simulink model "engine_throttle_control_eric_2"  (R2026a)
settings: Solver=VariableStepAuto
undefined symbols (not defined in the file or in its folder): constantsSTADPOLE
settings Model: Creator=Eric  LastModifiedBy=Eric

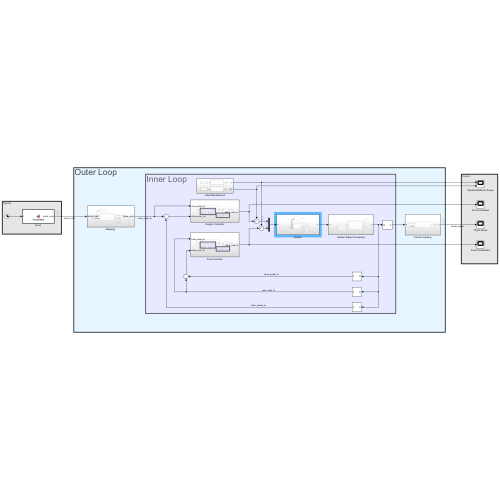
[thumbnail: Simulink's stored preview of the top-level diagram]
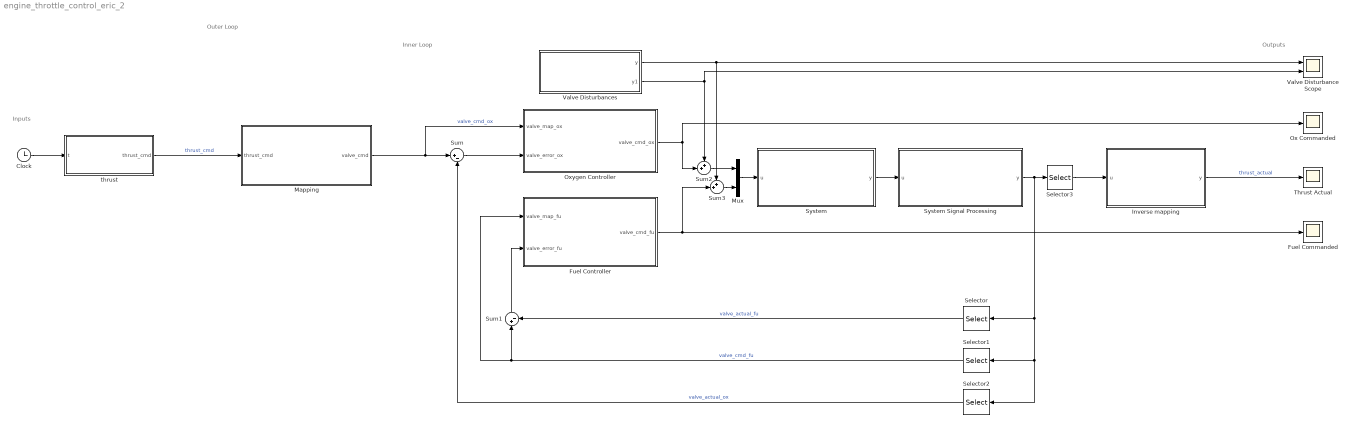
== system engine_throttle_control_eric_2 ==
  note: Inputs
  note: Outputs
  note: Outer Loop
  note: Inner Loop
  Clock : Clock
  Fuel Commanded : Scope
      settings: ActiveDisplayYMinimum=10.461022120017061  ActiveDisplayYMaximum=85.850800919846463  DataLoggingVariableName=ScopeData2
  Fuel Controller : Subsystem
  Inverse mapping : Subsystem
  Mapping : Subsystem
  Mux : Mux  Inputs=2
  Ox Commanded : Scope
      settings: ActiveDisplayYMinimum=6.6145825944924042  ActiveDisplayYMaximum=206.61458259449239  DataLoggingVariableName=ScopeData3
  Oxygen Controller : Subsystem
  Selector : Selector  InputPortWidth=6  IndexOptions=Index vector (dialog)  Indices=4  OutputSizes=1
  Selector1 : Selector  InputPortWidth=6  IndexOptions=Index vector (dialog)  Indices=3  OutputSizes=1
  Selector2 : Selector  InputPortWidth=6  IndexOptions=Index vector (dialog)  Indices=2  OutputSizes=1
  Selector3 : Selector  InputPortWidth=6  IndexOptions=Index vector (dialog)  Indices=1  OutputSizes=1
  Sum : Sum  Inputs=|+-
  Sum1 : Sum  Inputs=|+-
  Sum2 : Sum  Inputs=++|
  Sum3 : Sum  Inputs=++|
  System : Subsystem
  System Signal Processing : Subsystem
  Thrust Actual : Scope
      settings: ActiveDisplayYMinimum=-315.35197548585552  ActiveDisplayYMaximum=2620.6061100786883
  Valve Disturbance Scope : Scope  NumInputPorts=2
      settings: ActiveDisplayYMinimum=-2.4231337070144896  ActiveDisplayYMaximum=3.2939078653946221
  Valve Disturbances : Subsystem
  thrust : MATLAB Function  TreatAsAtomicUnit=on
  wires:
  Clock/1 -> thrust/1(t)
  Inverse mapping/1(y) -> Thrust Actual/1  "thrust_actual"
  thrust/1(thrust_cmd) -> Mapping/1(thrust_cmd)  "thrust_cmd"
  Sum/1 -> Oxygen Controller/2(valve_error_ox)
  Mapping/1(valve_cmd) -> Sum/1, Oxygen Controller/1(valve_map_ox)  "valve_cmd_ox"
  Oxygen Controller/1(valve_cmd_ox) -> Ox Commanded/1, Sum2/2
  System/1(y) -> System Signal Processing/1(u)
  System Signal Processing/1(y) -> Selector/1, Selector1/1, Selector2/1, Selector3/1
  Sum1/1 -> Fuel Controller/2(valve_error_fu)
  Fuel Controller/1(valve_cmd_fu) -> Sum3/2, Fuel Commanded/1
  Selector/1 -> Sum1/2  "valve_actual_fu"
  Selector1/1 -> Sum1/1, Fuel Controller/1(valve_map_fu)  "valve_cmd_fu"
  Selector2/1 -> Sum/2  "valve_actual_ox"
  Selector3/1 -> Inverse mapping/1(u)
  Sum2/1 -> Mux/1
  Valve Disturbances/2(y1) -> Sum2/1, Valve Disturbance Scope/2
  Sum3/1 -> Mux/2
  Valve Disturbances/1(y) -> Sum3/1, Valve Disturbance Scope/1
  Mux/1 -> System/1(u)

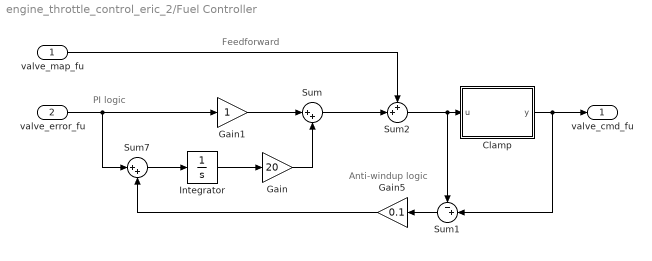
== system engine_throttle_control_eric_2/Fuel Controller ==
  note: PI logic
  note: Anti-windup logic
  note: Feedforward
  valve_map_fu : Inport
  valve_error_fu : Inport  Port=2
  Clamp : MATLAB Function  TreatAsAtomicUnit=on
  Gain : Gain  Gain=20
  Gain1 : Gain
  Gain5 : Gain  Gain=0.1
  Integrator : Integrator
  Sum : Sum  Inputs=|++
  Sum1 : Sum  Inputs=-+|
  Sum2 : Sum  Inputs=++|
  Sum7 : Sum  Inputs=|++
  valve_cmd_fu : Outport
  wires:
  Sum2/1 -> Clamp/1(u), Sum1/1
  Clamp/1(y) -> valve_cmd_fu/1, Sum1/2
  valve_map_fu/1 -> Sum2/1
  Sum1/1 -> Gain5/1
  Sum7/1 -> Integrator/1
  valve_error_fu/1 -> Sum7/1, Gain1/1
  Gain5/1 -> Sum7/2
  Gain/1 -> Sum/2
  Gain1/1 -> Sum/1
  Sum/1 -> Sum2/2
  Integrator/1 -> Gain/1

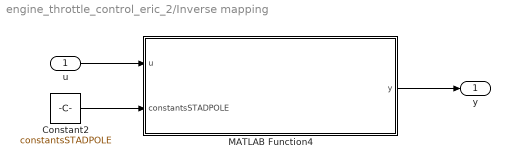
== system engine_throttle_control_eric_2/Inverse mapping ==
  u : Inport
  Constant2 : Constant  Value=constantsSTADPOLE  OutDataTypeStr=Bus: slBus1
  MATLAB Function4 : MATLAB Function  TreatAsAtomicUnit=on
  y : Outport
  wires:
  MATLAB Function4/1(y) -> y/1
  u/1 -> MATLAB Function4/1(u)
  Constant2/1 -> MATLAB Function4/2(constantsSTADPOLE)

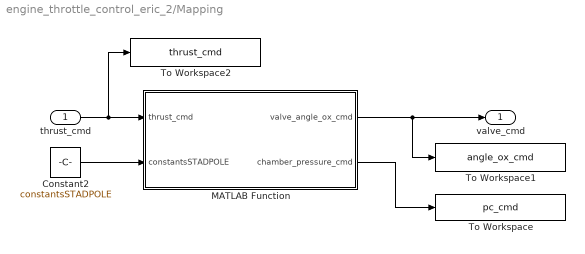
== system engine_throttle_control_eric_2/Mapping ==
  thrust_cmd : Inport
  Constant2 : Constant  Value=constantsSTADPOLE  OutDataTypeStr=Bus: slBus1
  MATLAB Function : MATLAB Function  TreatAsAtomicUnit=on
  To Workspace : ToWorkspace  VariableName=pc_cmd  SaveFormat=Timeseries  SampleTime=-1
  To Workspace1 : ToWorkspace  VariableName=angle_ox_cmd  SaveFormat=Timeseries  SampleTime=-1
  To Workspace2 : ToWorkspace  VariableName=thrust_cmd  SaveFormat=Timeseries  SampleTime=-1
  valve_cmd : Outport
  wires:
  MATLAB Function/1(valve_angle_ox_cmd) -> To Workspace1/1, valve_cmd/1
  thrust_cmd/1 -> To Workspace2/1, MATLAB Function/1(thrust_cmd)
  Constant2/1 -> MATLAB Function/2(constantsSTADPOLE)
  MATLAB Function/2(chamber_pressure_cmd) -> To Workspace/1

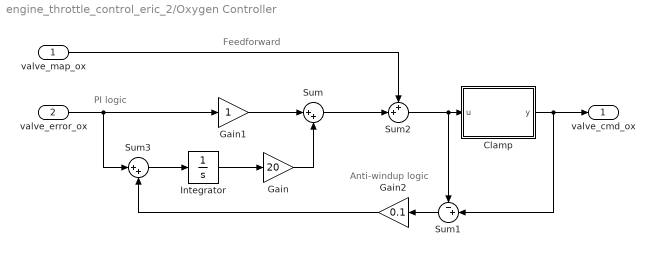
== system engine_throttle_control_eric_2/Oxygen Controller ==
  note: PI logic
  note: Anti-windup logic
  note: Feedforward
  valve_map_ox : Inport
  valve_error_ox : Inport  Port=2
  Clamp : MATLAB Function  TreatAsAtomicUnit=on
  Gain : Gain  Gain=20
  Gain1 : Gain
  Gain2 : Gain  Gain=0.1
  Integrator : Integrator
  Sum : Sum  Inputs=|++
  Sum1 : Sum  Inputs=-+|
  Sum2 : Sum  Inputs=++|
  Sum3 : Sum  Inputs=|++
  valve_cmd_ox : Outport
  wires:
  valve_error_ox/1 -> Sum3/1, Gain1/1
  Integrator/1 -> Gain/1
  Gain1/1 -> Sum/1
  Gain/1 -> Sum/2
  valve_map_ox/1 -> Sum2/1
  Sum3/1 -> Integrator/1
  Sum1/1 -> Gain2/1
  Gain2/1 -> Sum3/2
  Sum/1 -> Sum2/2
  Sum2/1 -> Clamp/1(u), Sum1/1
  Clamp/1(y) -> Sum1/2, valve_cmd_ox/1

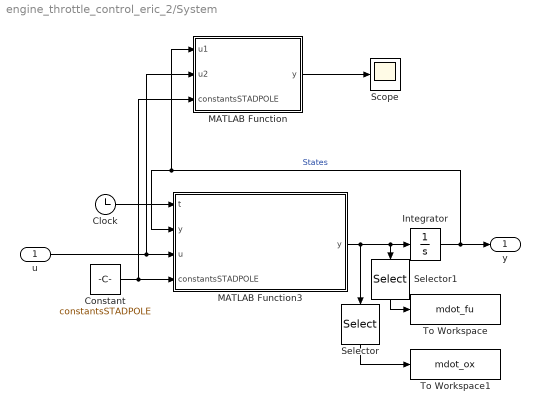
== system engine_throttle_control_eric_2/System ==
  u : Inport
  Clock : Clock
  Constant : Constant  Value=constantsSTADPOLE  OutDataTypeStr=Bus: slBus1
  Integrator : Integrator  InitialCondition=constantsSTADPOLE.init_cond
  MATLAB Function : MATLAB Function  TreatAsAtomicUnit=on
  MATLAB Function3 : MATLAB Function  TreatAsAtomicUnit=on
  Scope : Scope
      settings: DataLoggingVariableName=ScopeData4
  Selector : Selector  InputPortWidth=7  IndexOptions=Index vector (dialog)  Indices=1  OutputSizes=1
  Selector1 : Selector  InputPortWidth=7  IndexOptions=Index vector (dialog)  Indices=2  OutputSizes=1
  To Workspace : ToWorkspace  VariableName=mdot_fu  SaveFormat=Timeseries  SampleTime=-1
  To Workspace1 : ToWorkspace  VariableName=mdot_ox  SaveFormat=Timeseries  SampleTime=-1
  y : Outport
  wires:
  MATLAB Function3/1(y) -> Selector/1, Selector1/1, Integrator/1
  u/1 -> MATLAB Function/2(u2), MATLAB Function3/3(u)
  Integrator/1 -> MATLAB Function3/2("y "), MATLAB Function/1(u1), y/1  "States"
  Constant/1 -> MATLAB Function/3(constantsSTADPOLE), MATLAB Function3/4(constantsSTADPOLE)
  Clock/1 -> MATLAB Function3/1(t)
  Selector/1 -> To Workspace1/1
  Selector1/1 -> To Workspace/1
  MATLAB Function/1(y) -> Scope/1

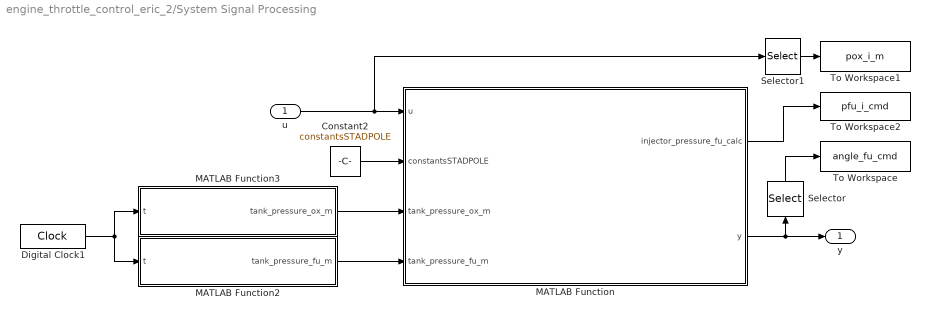
== system engine_throttle_control_eric_2/System Signal Processing ==
  u : Inport
  Constant2 : Constant  Value=constantsSTADPOLE  OutDataTypeStr=Bus: slBus1
  Digital Clock1 : DigitalClock
  MATLAB Function : MATLAB Function  TreatAsAtomicUnit=on
  MATLAB Function2 : MATLAB Function  TreatAsAtomicUnit=on
  MATLAB Function3 : MATLAB Function  TreatAsAtomicUnit=on
  Selector : Selector  InputPortWidth=6  IndexOptions=Index vector (dialog)  Indices=3  OutputSizes=1
  Selector1 : Selector  InputPortWidth=7  IndexOptions=Index vector (dialog)  Indices=4  OutputSizes=1
  To Workspace : ToWorkspace  VariableName=angle_fu_cmd  SaveFormat=Timeseries  SampleTime=-1
  To Workspace1 : ToWorkspace  VariableName=pox_i_m  SaveFormat=Timeseries  SampleTime=-1
  To Workspace2 : ToWorkspace  VariableName=pfu_i_cmd  SaveFormat=Timeseries  SampleTime=-1
  y : Outport
  wires:
  MATLAB Function/2(y) -> y/1, Selector/1
  Constant2/1 -> MATLAB Function/2(constantsSTADPOLE)
  MATLAB Function3/1(tank_pressure_ox_m) -> MATLAB Function/3(tank_pressure_ox_m)
  Digital Clock1/1 -> MATLAB Function3/1(t), MATLAB Function2/1(t)
  MATLAB Function2/1(tank_pressure_fu_m) -> MATLAB Function/4(tank_pressure_fu_m)
  Selector/1 -> To Workspace/1
  Selector1/1 -> To Workspace1/1
  u/1 -> Selector1/1, MATLAB Function/1(u)
  MATLAB Function/1(injector_pressure_fu_calc) -> To Workspace2/1

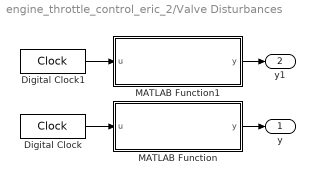
== system engine_throttle_control_eric_2/Valve Disturbances ==
  Digital Clock : DigitalClock
  Digital Clock1 : DigitalClock
  MATLAB Function : MATLAB Function  TreatAsAtomicUnit=on
  MATLAB Function1 : MATLAB Function  TreatAsAtomicUnit=on
  y : Outport
  y1 : Outport  Port=2
  wires:
  MATLAB Function/1(y) -> y/1
  Digital Clock/1 -> MATLAB Function/1(u)
  MATLAB Function1/1(y) -> y1/1
  Digital Clock1/1 -> MATLAB Function1/1(u)

== matlab function engine_throttle_control_eric_2/Fuel Controller/Clamp ==
  data: u input; y output
function y = sat(u)

if u < 0
    y = 0;

elseif 90 < u
    y = 90;

else
    y = u;

end

== matlab function engine_throttle_control_eric_2/Mapping/MATLAB Function ==
  data: thrust_cmd input; valve_angle_ox_cmd output; constantsSTADPOLE input; chamber_pressure_cmd output
function [valve_angle_ox_cmd, chamber_pressure_cmd] = thrust_to_valve_mapping(thrust_cmd, constantsSTADPOLE)

throat_area = constantsSTADPOLE.a_t;                % [m^2]
thrust_coeff = constantsSTADPOLE.c_f;               % [unitless]
char_vel = constantsSTADPOLE.c_star;                % [m/s]
of_ratio = constantsSTADPOLE.OF_target;             % [unitless]
rho_ox = constantsSTADPOLE.dens_o;                  % [kg/m^3]
discharge_coeff_ox = constantsSTADPOLE.d_coeff_ox;  % [unitless],  -------------Random value just to get the code to run
orifice_area_ox = constantsSTADPOLE.a_i_o;          % [m^2],  -------------Random value just to get the code to run
rho_water = constantsSTADPOLE.dens_w;               % [kg/m^3]

% Valve Coefficient Calculations 
chamber_pressure_cmd = thrust_cmd / (throat_area * thrust_coeff);   % [Pa]
massflow_tot_cmd = chamber_pressure_cmd * throat_area / char_vel;   % [kg/s]
massflow_ox_cmd = massflow_tot_cmd * of_ratio / (of_ratio + 1);     % [kg/s]
friction_pressure_drop_ox = 96402.2 * massflow_ox_cmd^2;
injector_pressure_ox_cmd = chamber_pressure_cmd + (massflow_ox_cmd ^ 2) / (2 * rho_ox * (discharge_coeff_ox * orifice_area_ox) ^ 2); % [Pa]
%% assume 550 PSI for tank 
valve_coeff_ox_cmd = massflow_ox_cmd * sqrt(max(1 / (rho_ox * rho_water * (3.792E6 - friction_pressure_drop_ox - injector_pressure_ox_cmd)), 0)); % [m^3.5/kg^0.5]

% NEED VALVE COEFFICIENT TO VALVE ANGLE FUNCTION

valve_angle_ox_cmd = CoefficientToAngle(valve_coeff_ox_cmd);

== matlab function engine_throttle_control_eric_2/thrust ==
  data: t input; thrust_cmd output
function thrust_cmd = ThrustPlant(t)
% %THRUSTPLANT 
% %   random plant function for the thrust in the engine
% if t < 2
%     thrust_cmd = 0; %[N]
% elseif mod(t,5) < 3
%     thrust_cmd = 1500;
% else
%     thrust_cmd = 1500 - 500 * sin(mod(t,5) * pi / 2);
% 
% end
% %cosint(t*pi/180);

    % if t < 5.0
    %     thrust_cmd = 2000; % [N] Step 1: 0s to 5s
    % else
    %     thrust_cmd = -400 * t + 4000;    % [N] Step 2: 5s to 10s
    % end

    % if t < 3.0
    %     thrust_cmd = 2000;
    % elseif 3 <= t && t <= 6
    %     thrust_cmd = 1000;
    % else
    %     thrust_cmd = 200 * t - 200;
    % end

    thrust_cmd = 500 * cos(t) + 1500;
end

== matlab function engine_throttle_control_eric_2/System Signal Processing/MATLAB Function3 ==
  data: t input; tank_pressure_ox_m output
function tank_pressure_ox_m = oxygen_tank_pressure(t)

% Simulate oxygen tank pressure, for now, assume constant at 550 psi or 
% 3.792 MPa

tank_pressure_ox_m = 3.792E6; % [Pa]

== matlab function engine_throttle_control_eric_2/System Signal Processing/MATLAB Function2 ==
  data: t input; tank_pressure_fu_m output
function tank_pressure_fu_m = fuel_tank_pressure(t)

% Simulate fuel tank pressure, for now, assume constant at 550 psi or 3.792
% MPa

tank_pressure_fu_m = 3.792E6; % [MPa]

== matlab function engine_throttle_control_eric_2/System/MATLAB Function3 ==
  data: t input; y input; u input; y output; constantsSTADPOLE input
function y = system_model(t, y, u, constantsSTADPOLE)
    
    % y(1)' = time rate of mass flow oxygen [kg/s^2]
    % y(2)' = time rate of mass flow fuel [kg/s^2]
    % y(3)' = time rate of chamber pressure [Pa/s]
    % y(4)' = time rate of oxygen injector press [Pa/s]
    % y(5)' = time rate of fuel injector press [Pa/s]
    % y(6)' = time rate of oxygen pressure at valve [Pa/s]
    % y(7)' = time rate of fuel pressure at valve [Pa/s]

    % y(1) = mass flow oxygen across pipe [kg/s]
    % y(2) = mass flow fuel across pipe [kg/s]
    % y(3) = chamber pressure [Pa]
    % y(4) = oxygen pressure at inj [Pa]
    % y(5) = fuel pressure at inj [Pa]
    % y(6) = oxygen pressure at valve [Pa]
    % y(7) = fuel pressure at valve [Pa]
    
    a_t= constantsSTADPOLE.a_t ; % [m^2], throat area
    
    dens_o = constantsSTADPOLE.dens_o; % [kg/m^3], liquid oxygen density, at 90 K and 1 atm
    dens_f = constantsSTADPOLE.dens_f ; % [kg/m^3], fuel density, at 293 K and 1 atm
    dens_w = constantsSTADPOLE.dens_w ; % [kg/m^3], water density
    g = constantsSTADPOLE.g ; % [m/s^2], acceleration due to gravity
    a_i_o = constantsSTADPOLE.a_i_o; % [m^2] area injector ox
    a_i_f = constantsSTADPOLE.a_i_f ; % [m^2] area injector fuel
    r = constantsSTADPOLE.r ; % [J/kg-K], specific gas constant of exhaust (molecular weight 18.8 g/mol)
    c_star = constantsSTADPOLE.c_star ; % [m/s] characteristic velocity
    of = constantsSTADPOLE.OF_target;

    c_fric = 0.03; % [unitless], line friction coefficient
    c_d_o = constantsSTADPOLE.d_coeff_ox; % [unitless], oxygen injector coefficient
    c_d_f = constantsSTADPOLE.d_coeff_fu; % [unitless], fuel injector coefficient
    l_eq_o = 7 * 0.0254; % [m], oxygen equivalent line length 
    l_eq_f = 7 * 0.0254; % [m], fuel equivalent line length 
    l_o = 120 * 0.0254; % [m], oxygen line length
    l_f = 60 * 0.0254; % [m], fuel line length
    d = (0.5 - 2 * 0.065) * 0.0254; % [m], line diameter
    v_c = 1.103170594 * 1e-3; % [m^3], chamber volume
    a_l = pi * (d / 2) ^ 2; % [m^2], line area
  
    v_l_o = a_l * l_o;
    v_l_f = a_l * l_f;
    t_o = 90; 
    t_f = 293;

    % Assume constant?
    c_v_o = AngleToCoefficient(u(1,1));  % 1.231e-06; [m^3.5/kg^0.5], oxygen valve coefficient
    c_v_f = AngleToCoefficient(u(2,1));  % 1.231e-06; [], fuel valve coefficient
    p_tank_o = 3.792E6; % [Pa]
    p_tank_f = 3.792E6; % [Pa]
    t_c = 3570; % [K], chamber temperature
    

    del_p_i_o = 1 / (2 * dens_o * (c_d_o * a_i_o) ^ 2); 
    del_p_l_o = 96402.2;
    del_p_i_f = 1 / (2 * dens_f * (c_d_f * a_i_f) ^ 2); 
    del_p_l_f = 2082581.1;
    

    % Momentum equations
    % massflow across pipe
    % mdot_pipe_ox = (y(4) - y(3) - del_p_l_o * y(1) * sqrt(y(1)^2 + 1e-6)) * a_l / l_o;
    % mdot_pipe_fu = (y(5) - y(3) - del_p_l_f * y(2) * sqrt(y(2)^2 + 1e-6)) * a_l / l_f;
    mddot_pipe_ox = (y(6) - y(4) - del_p_l_o * y(1) * sqrt(y(1)^2 + 1e-6)) * a_l / l_o;
    mddot_pipe_fu = (y(7) - y(5) - del_p_l_f * y(2) * sqrt(y(2)^2 + 1e-6)) * a_l / l_f;

    % Valve massflows
    ValveOX = dens_o * dens_w * (p_tank_o - y(6));
    ValveFU = dens_f * dens_w * (p_tank_f - y(7));
    mdot_valve_ox = c_v_o * ValveOX / sqrt(abs(ValveOX) + 1e2);
    mdot_valve_fu = c_v_f * ValveFU / sqrt(abs(ValveFU) + 1e2);

    % Injector massflows
    InjectorOX = 2 * dens_o *(y(4)-y(3));
    InjectorFU = 2 * dens_f * (y(5)-y(3));
    mdot_inj_ox = c_d_o * a_i_o * InjectorOX / sqrt(abs(InjectorOX)+1e2);
    mdot_inj_fu = c_d_f * a_i_f * InjectorFU / sqrt(abs(InjectorFU)+1e2);

    % Pressure at the end of the valve
    valve_ox_dot = 1e9 / (v_l_o * dens_o) * (mdot_valve_ox - y(1));
    valve_fu_dot = 1e9 / (v_l_f * dens_f) * (mdot_valve_fu - y(2));

    inj_ox_dot = 1e9 / (v_l_o*dens_o) * (y(1) - mdot_inj_ox);
    inj_fu_dot = 1e9 / (v_l_f*dens_f) * (y(2) - mdot_inj_fu);

    % Chamber Pressure equations
    pdot_chamber = (r * t_c / v_c) * (mdot_inj_ox + mdot_inj_fu - a_t * y(3) / c_star);

    % Final system
    y = [mddot_pipe_ox; mddot_pipe_fu; pdot_chamber; inj_ox_dot; inj_fu_dot; valve_ox_dot; valve_fu_dot];

end

== matlab function engine_throttle_control_eric_2/Inverse mapping/MATLAB Function4 ==
  data: u input; y output; constantsSTADPOLE input
function y = valve_to_thrust_mapping(u, constantsSTADPOLE)

throat_area = constantsSTADPOLE.a_t; % [m^2]
thrust_coeff = constantsSTADPOLE.c_f; % [unitless]

y = u * thrust_coeff * throat_area;

== matlab function engine_throttle_control_eric_2/System Signal Processing/MATLAB Function ==
  data: injector_pressure_fu_calc output; u input; y output; constantsSTADPOLE input; tank_pressure_ox_m input; tank_pressure_fu_m input
function [injector_pressure_fu_calc, y] = sensor_function(u, constantsSTADPOLE, tank_pressure_ox_m, tank_pressure_fu_m)

% *************************************************************************
% Constants

of_ratio = constantsSTADPOLE.OF_target; % [unitless]
rho_ox = constantsSTADPOLE.dens_o; % [kg/m^3]
rho_fu = constantsSTADPOLE.dens_f; % [kg/m^3]
discharge_coeff_ox = constantsSTADPOLE.d_coeff_ox; % [unitless],  -------------Random value just to get the code to run
discharge_coeff_fu = constantsSTADPOLE.d_coeff_fu; % [unitless],  -------------Random value just to get the code to run
orifice_area_ox = constantsSTADPOLE.a_i_o; % [m^2],  -------------Random value just to get the code to run
orifice_area_fu = constantsSTADPOLE.a_i_f; % [m^2],  -------------Random value just to get the code to run
throat_area = constantsSTADPOLE.a_t; % [m^2]
char_vel = constantsSTADPOLE.c_star; % [m/s]

% 150 psi at max thrust, quarter at 50%
rho_water = constantsSTADPOLE.dens_w; % [kg/m^3]

% *************************************************************************
% Inputs

% u(1) = mass flow oxygen across pipe [kg/s]
% u(2) = mass flow fuel across pipe [kg/s]
% u(3) = chamber pressure [Pa]
% u(4) = oxygen pressure at inj [Pa]
% u(5) = fuel pressure at inj [Pa]
% u(6) = oxygen pressure at valve [Pa]
% u(7) = fuel pressure at valve [Pa]

chamber_pressure_m = u(3);
injector_pressure_ox_m = u(4);
injector_pressure_fu_m = u(5);

% *************************************************************************
% Fuel Valve command

% Calculates fuel valve command based on oxygen injector pressure and
% chamber pressure

% Valve coefficient equations
delta_p_injector_ox_calc = max(injector_pressure_ox_m - chamber_pressure_m, 0); % [Pa]
term_1 = sqrt(2 * delta_p_injector_ox_calc * rho_ox); % [kg/m^2-s]
massflow_ox_calc = discharge_coeff_ox * orifice_area_ox * term_1; % [kg/s]
massflow_fu_calc = massflow_ox_calc / of_ratio; % [kg/s]
injector_pressure_fu_calc = chamber_pressure_m + (massflow_fu_calc ^ 2) / (2 * rho_fu * (discharge_coeff_fu * orifice_area_fu) ^ 2); % [Pa]
friction_pressure_drop_fu = massflow_fu_calc^2 * 2082581.1;
valve_coeff_fu_cmd = massflow_fu_calc *  sqrt(max(1 / (rho_fu * rho_water * (tank_pressure_fu_m - friction_pressure_drop_fu - injector_pressure_fu_calc)), 0)); % [m^3.5/kg^0.5]

% NEED COEFFICIENT TO ANGLE MAPPING

% *************************************************************************
% Fuel Valve actual

delta_p_injector_fu_calc = max(injector_pressure_fu_m - chamber_pressure_m, 0); % [Pa]
term_2 = sqrt(2 * delta_p_injector_fu_calc * rho_fu); % [kg/m^2-s]
massflow_fu_calc2 = discharge_coeff_fu * orifice_area_fu * term_2; % [kg/s]
valve_coeff_fu_actual = massflow_fu_calc2 *  sqrt(max(1 / (rho_fu * rho_water * (tank_pressure_fu_m - friction_pressure_drop_fu - injector_pressure_fu_m)), 0)); % [m^3.5/kg^0.5]

% *************************************************************************
% Oxygen Valve actual

% massflow_tot_m = chamber_pressure_m * throat_area / char_vel; % [kg/s]
% massflow_ox_m = massflow_tot_m * of_ratio / (of_ratio + 1); % [kg/s]
friction_pressure_drop_ox = 96402.2 * massflow_ox_calc^2;
valve_coeff_ox_actual = massflow_ox_calc * sqrt(max(1 / (rho_ox * rho_water * (tank_pressure_ox_m - friction_pressure_drop_ox - injector_pressure_ox_m)), 0)); % [m^3.5/kg^0.5]

% *************************************************************************
% Outputs

valve_angle_ox_actual = CoefficientToAngle(valve_coeff_ox_actual); 
valve_angle_fu_cmd = CoefficientToAngle(valve_coeff_fu_cmd); 
valve_angle_fu_actual = CoefficientToAngle(valve_coeff_fu_actual);

y = [chamber_pressure_m; valve_angle_ox_actual; valve_angle_fu_cmd; valve_angle_fu_actual; tank_pressure_ox_m; tank_pressure_fu_m];

== matlab function engine_throttle_control_eric_2/Oxygen Controller/Clamp ==
  data: u input; y output
function y = sat(u)

if u < 0
    y = 0;

elseif 90 < u
    y = 90;

else
    y = u;

end

== matlab function engine_throttle_control_eric_2/Valve Disturbances/MATLAB Function ==
  data: u input; y output
function y = valve_disturbance_ox(u)

y = 0*randn(1);

== matlab function engine_throttle_control_eric_2/Valve Disturbances/MATLAB Function1 ==
  data: u input; y output
function y = valve_disturbance_fu(u)

y = 0*randn(1);

== matlab function engine_throttle_control_eric_2/System/MATLAB Function ==
  data: u1 input; y output; u2 input; constantsSTADPOLE input
function y = fcn(u1, u2, constantsSTADPOLE)

% u1(1) = mass flow oxygen across pipe [kg/s]
% u1(2) = mass flow fuel across pipe [kg/s]
% u1(3) = chamber pressure [Pa]
% u1(4) = oxygen pressure at inj [Pa]
% u1(5) = fuel pressure at inj [Pa]
% u1(6) = oxygen pressure at valve [Pa]
% u1(7) = fuel pressure at valve [Pa]

% u2(1) = oxygen valve coefficient
% u2(2) = fuel valve coefficient

dens_o = constantsSTADPOLE.dens_o; % [kg/m^3], liquid oxygen density, at 90 K and 1 atm
dens_f = constantsSTADPOLE.dens_f ; % [kg/m^3], fuel density, at 293 K and 1 atm
a_i_o = constantsSTADPOLE.a_i_o; % [m^2] area injector ox
a_i_f = constantsSTADPOLE.a_i_f ; % [m^2] area injector fuel
c_d_o = constantsSTADPOLE.d_coeff_ox; % [unitless], oxygen injector coefficient
c_d_f = constantsSTADPOLE.d_coeff_fu; % [unitless], fuel injector coefficient

p_tank_o = 3.7921E+06;
p_tank_f = 3.7921E+06;

mdot_ox_inj = c_d_o * a_i_o * sqrt(2 * dens_o * (u1(4) - u1(3)));
mdot_fu_inj = c_d_f * a_i_f * sqrt(2 * dens_f * (u1(5) - u1(3)));

mdot_ox_valve = AngleToCoefficient(u2(1)) * sqrt(2 * dens_o * (p_tank_o - u1(6)));
mdot_fu_valve = AngleToCoefficient(u2(2)) * sqrt(2 * dens_f * (p_tank_f - u1(7)));

y = [mdot_ox_inj, mdot_fu_inj, mdot_ox_valve, mdot_fu_valve];
